simulink model "FBStateFlow"  (R2018b)
settings: Solver=FixedStepAuto  StartTime=0.0  StopTime=10.0  RelTol=1e-3
values from neighbouring files (symbols this model uses):
  done_code = uint8(5)    [setup.m]
  error_code = uint8(6)    [setup.m]
  execute_code = uint8(3)    [setup.m]
  idle_code = uint8(1)    [setup.m]
  init_code = uint8(0)    [setup.m]
  read_input_code = uint8(2)    [setup.m]
  write_output_code = uint8(4)    [setup.m]
settings Model: Creator=hiterd  LastModifiedBy=gauthamsm
settings SFSimCC: SimUseLocalCustomCode=off
settings RTWCC: RTWUseLocalCustomCode=off

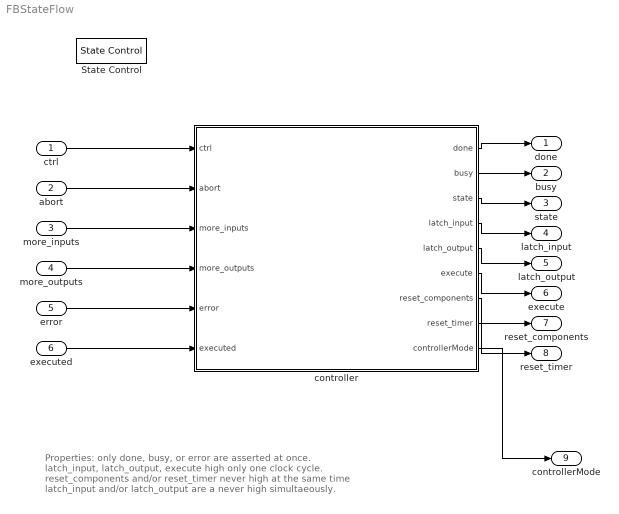
== system FBStateFlow ==
  note: Properties:
      | only done, busy, or error are asserted at once.
      | latch_input, latch_output, execute high only one clock cycle.
      | reset_components and/or reset_timer never high at the same time latch_input and/or latch_output are a never high simultaeously.
  ctrl : Inport  OutDataTypeStr=boolean
  abort : Inport  Port=2  OutDataTypeStr=boolean
  more_inputs : Inport  Port=3  OutDataTypeStr=boolean
  more_outputs : Inport  Port=4  OutDataTypeStr=boolean
  error : Inport  Port=5  OutDataTypeStr=boolean
  executed : Inport  Port=6  OutDataTypeStr=boolean
  State Control : StateControl  StateControl=Synchronous
  controller : Stateflow chart  TreatAsAtomicUnit=on
  done : Outport
  busy : Outport  Port=2
  state : Outport  Port=3
  latch_input : Outport  Port=4
  latch_output : Outport  Port=5
  execute : Outport  Port=6
  reset_components : Outport  Port=7
  reset_timer : Outport  Port=8
  "controllerMode " : Outport  Port=9
  wires:
  controller/8(reset_timer) -> reset_timer/1
  controller/2(busy) -> busy/1
  controller/4(latch_input) -> latch_input/1
  controller/5(latch_output) -> latch_output/1
  executed/1 -> controller/6(executed)
  controller/7(reset_components) -> reset_components/1
  controller/1(done) -> done/1
  more_outputs/1 -> controller/4(more_outputs)
  controller/6(execute) -> execute/1
  error/1 -> controller/5(error)
  controller/3(state) -> state/1
  more_inputs/1 -> controller/3(more_inputs)
  abort/1 -> controller/2(abort)
  ctrl/1 -> controller/1(ctrl)
  controller/9(controllerMode) -> "controllerMode "/1

== stateflow chart FBStateFlow/controller ==
  settings: stateMachineType=MOORE_MACHINE  executeAtInitialization=1  initializeOutput=1
  state INIT
    done = false;
    busy = false;
    state = init_code;
    latch_input = false;
    latch_output = false;
    execute = false;
    reset_components = true;
    reset_timer = true;
  state IDLE
    done = false;
    busy = false;
    state = idle_code;
    latch_input = false;
    latch_output = false;
    execute = false;
    reset_components = true;
    reset_timer = false;
  state READ_INPUT
    state read
      done = false;
      busy = true;
      state = read_input_code;
      latch_input = true;
      latch_output = false;
      execute = false;
      reset_components = false;
      reset_timer = false;
    state not_read
      done = false;
      busy = false;
      state = read_input_code;
      latch_input = false;
      latch_output = false;
      execute = false;
      reset_components = false;
      reset_timer = false;
    (default) -> read
    read -> not_read
  state EXECUTE
    state execute
      done = false;
      busy = true;
      state = execute_code;
      latch_input = false;
      latch_output = false;
      execute = true;
      reset_components = false;
      reset_timer = false;
    state complete
      done = false;
      busy = false;
      state = execute_code;
      latch_input = false;
      latch_output = false;
      execute = false;
      reset_components = false;
      reset_timer = false;
    (default) -> execute
    execute -> complete : [executed]
  state ERROR
    done = false;
    busy = false;
    state = error_code;
    latch_input = false;
    latch_output = false;
    execute = false;
    reset_components = false;
    reset_timer = false;
  state WRITE_OUTPUT
    state write
      done = false;
      busy = true;
      state = write_output_code;
      latch_input = false;
      latch_output = true;
      execute = false;
      reset_components = false;
      reset_timer = false;
    state not_write
      done = false;
      busy = false;
      state = write_output_code;
      latch_input = false;
      latch_output = false;
      execute = false;
      reset_components = false;
      reset_timer = false;
    (default) -> write
    write -> not_write
  state DONE
    done = true;
    busy = false;
    state = done_code;
    latch_input = false;
    latch_output = false;
    execute = false;
    reset_components = false;
    reset_timer = false;
  not_read -> (junction 41) : [ctrl]
  not_write -> (junction 44) : [ctrl]
  complete -> WRITE_OUTPUT : [ctrl]
  (default) -> INIT
  (junction 35) -> INIT [order 1] : [abort]
  DONE -> INIT : [ctrl]
  INIT -> IDLE
  (junction 35) -> IDLE [order 2]
  ERROR -> (junction 35) : [ctrl]
  IDLE -> READ_INPUT : [ctrl]
  READ_INPUT -> (junction 68)
  (junction 41) -> READ_INPUT [order 1] : [more_inputs]
  (junction 41) -> EXECUTE [order 2]
  EXECUTE -> (junction 68)
  (junction 68) -> ERROR : [error]
  WRITE_OUTPUT -> (junction 68)
  (junction 44) -> WRITE_OUTPUT [order 1] : [more_outputs]
  (junction 44) -> DONE [order 2]
  data: ctrl input boolean; abort input boolean; done output boolean; more_inputs input boolean; more_outputs input boolean; error input boolean; executed input boolean; busy output boolean; state output uint8; latch_input output boolean; latch_output output boolean; execute output boolean; reset_components output boolean; reset_timer output boolean; idle_code parameter uint8; init_code parameter uint8; read_input_code parameter uint8; execute_code parameter uint8; write_output_code parameter uint8; done_code parameter uint8; error_code parameter uint8; controllerMode output Enum: controllerModeType
